simulink model "i_isled"  (R2019b)
settings: Solver=VariableStepAuto  StartTime=0.0  StopTime=t_final  MaxStep=0.00001  RelTol=1e-3
values from neighbouring files (symbols this model uses):
  K1 = 3 + .1*(2*rand()-1)    [I_regul.m]
  Ki = Kia*T0    (= 0.01)    [I_regul.m]
  Kia = 1/(2*Tu*K1)    [I_regul.m]
  T0 = T1    [I_regul.m]
  T1 = .1 + .01*(2*rand()-1)    [I_regul.m]
settings Model: Creator=Anton Mayorov  LastModifiedBy=bedla
settings DataIOCC: ReturnWorkspaceOutputs=off
settings DebuggingCC: ArithmeticOperatorsInVariantConditions=warning
settings SFSimCC: SimUseLocalCustomCode=off  CustomCodeUndefinedFunction=UseInterfaceOnly
settings RTWCC: RTWUseLocalCustomCode=off

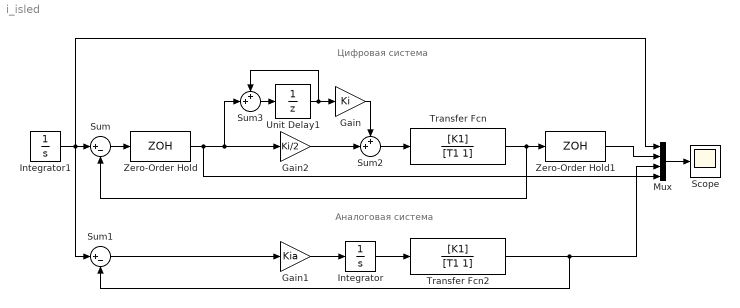
== system i_isled ==
  note: Аналоговая система
  note: Цифровая система
  Gain : Gain  Gain=Ki
  Gain1 : Gain  Gain=Kia
  Gain2 : Gain  Gain=Ki/2
  Integrator : Integrator
  Integrator1 : Integrator  InitialCondition=1
  Mux : Mux
  Scope : Scope
  Sum : Sum  Inputs=|+-
  Sum1 : Sum  Inputs=|+-
  Sum2 : Sum  Inputs=++|
  Sum3 : Sum  Inputs=++|
  Transfer Fcn : TransferFcn  Numerator=[K1]  Denominator=[T1 1]
  Transfer Fcn2 : TransferFcn  Numerator=[K1]  Denominator=[T1 1]
  Unit Delay1 : UnitDelay  SampleTime=-1  HasFrameUpgradeWarning=on
  Zero-Order Hold : ZeroOrderHold  SampleTime=T0
  Zero-Order Hold1 : ZeroOrderHold  SampleTime=T0
  wires:
  Mux/1 -> Scope/1
  Transfer Fcn/1 -> Zero-Order Hold1/1, Sum/2
  Sum/1 -> Zero-Order Hold/1
  Integrator1/1 -> Sum1/1, Mux/1, Sum/1
  Sum1/1 -> Gain1/1
  Transfer Fcn2/1 -> Mux/3, Sum1/2
  Gain1/1 -> Integrator/1
  Zero-Order Hold1/1 -> Mux/2
  Integrator/1 -> Transfer Fcn2/1
  Sum2/1 -> Transfer Fcn/1
  Gain2/1 -> Sum2/2
  Zero-Order Hold/1 -> Sum3/2, Gain2/1, Mux/4
  Gain/1 -> Sum2/1
  Sum3/1 -> Unit Delay1/1
  Unit Delay1/1 -> Gain/1, Sum3/1
